simulink model "Depression"  (Simulink 6.3)
settings: Solver=ode23s  StartTime=0  StopTime=3500  MaxStep=0.5  RelTol=1e-3
undefined symbols (not defined in the file or in its folder): sigbuilder_block
Description:
  | This is a model of depression in synapses
settings Model: Creator=chchlee  LastModifiedBy=Owner  ExtModeAutoUpdateStatusClock=off
settings DataIOCC: SignalLoggingName=sigsOut
settings OptimizationCC: InlineInvariantSignals=on
settings DebuggingCC: SolverPrmCheckMsg=none
settings HardwareCC: TargetUnknown=on
settings GRTTargetCC: ModelReferenceCompliant=off  MatFileLogging=off

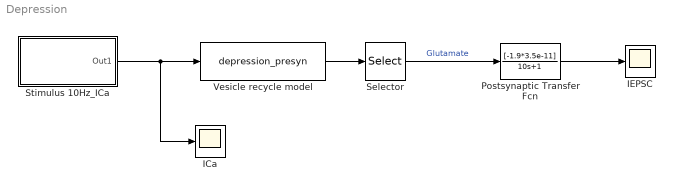
== system Depression ==
  ICa : Scope
      settings: YMin=-67.5  YMax=-63  SaveName=ScopeData3
  IEPSC : Scope
      settings: YMin=-2.2e-006  YMax=-1.04998e-038  SaveName=sim_depression10Hz  DataFormat=Array
  Postsynaptic Transfer Fcn : TransferFcn  Numerator=[-1.9*3.5e-11]  Denominator=[10 1]
  Selector : Selector  Elements=[4]  InputPortWidth=4
  Stimulus 10Hz_ICa : Subsystem
  Vesicle recycle model : S-Function  FunctionName=depression_presyn
  wires:
  Selector/1 -> Postsynaptic Transfer Fcn/1  "Glutamate"
  Vesicle recycle model/1 -> Selector/1
  Stimulus 10Hz_ICa/1(Out1) -> ICa/1, Vesicle recycle model/1
  Postsynaptic Transfer Fcn/1 -> IEPSC/1

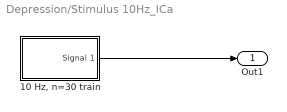
== system Depression/Stimulus 10Hz_ICa ==
  "10 Hz, n=30 train" : Subsystem  Tag=STV Subsys  LoadFcn=sigbuilder_block('load');  StartFcn=sigbuilder_block('start');  StopFcn=sigbuilder_block('stop');  ClipboardFcn=sigbuilder_block('clipboard');  mask(Sigbuilder block){}
      mask help: Sigbuilder GUI
      mask init:
      | if ~strcmp(get_param(bdroot(gcbh),'SimulationStatus'),'stopped') tuvar = sigbuilder_block('maskInit'); end
      settings: CopyFcn=sigbuilder_block('copy');  DeleteFcn=sigbuilder_block('delete');  ModelCloseFcn=sigbuilder_block('modelClose');  PreSaveFcn=sigbuilder_block('preSave');  NameChangeFcn=sigbuilder_block('namechange');  OpenFcn=sigbuilder_block('open',[-3 25.5 768 498 ]);  CloseFcn=sigbuilder_block('close');
      mask Display: plot(0,0,100,100,[10,10,40,40,10],[80,20,20,80,80],[40,10],[50,50], [40,27,10],[65,72,56],[40,25,25,10],[28,28,43,43]);
  Out1 : Outport
  wires:
  "10 Hz, n=30 train"/1(Signal 1) -> Out1/1

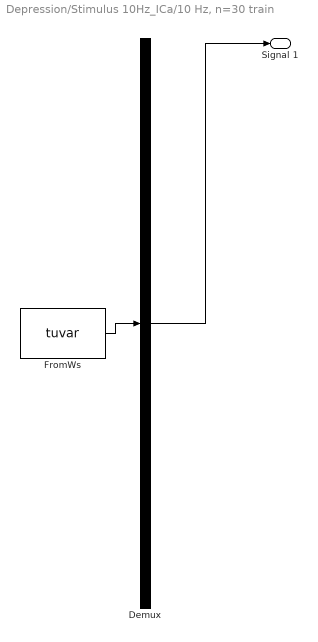
== system Depression/Stimulus 10Hz_ICa/10 Hz, n=30 train ==
  Demux : Demux  Tag=STV Demux  Outputs=1
  FromWs : FromWorkspace  Tag=STV FromWs  VariableName=tuvar  SampleTime=0  SigBuilderData=DataTag0  VnvData=DataTag1
      SigBuilderData=|
      | channels.label = 'Signal 1'
      | channels.allXData = {[0 100 100 101 101 200 200 201 201 300 300 301 301 400 400 401 401 500 500 501 501 600 600 601 601 700 700 701 701 800 800 801 801 900 900 901 901 1000 1000 1001 1001 1100 1100 1101 1101 1200 1200 1201 1201 1300 1300 1301 1301 1400 1400 1401 1401 1500 1500 1501 1501 1600 1600 1601 1601 1700 1700 1701 1701 1800 1800 1801 1801 1900 1900 1901 1901 2000 2000 2001 2001 2100 2100 2101 2101 2200 2200 2201 2201 2300 2300 2301 2301 2400 2400 2401 2401 2500 2500 2501 2501 2600 2600 2601 2601 2700 2700 2701 2701 2800 2800 2801 2801 2900 2900 2901 2901 3000 3000 3001 3001 3100 3100 3101 3101 3200 3300]}
      | channels.allYData = {[0 0 1 1 0 0 1 1 0 0 1 1 0 0 1 1 0 0 1 1 0 0 1 1 0 0 1 1 0 0 1 1 0 0 1 1 0 0 1 1 0 0 1 1 0 0 1 1 0 0 1 1 0 0 1 1 0 0 1 1 0 0 1 1 0 0 1 1 0 0 1 1 0 0 1 1 0 0 1 1 0 0 1 1 0 0 1 1 0 0 1 1 0 0 1 1 0 0 1 1 0 0 1 1 0 0 1 1 0 0 1 1 0 0 1 1 0 0 1 1 0 0 0 0 0 0 0]}
      | dataSet.timeRange = [0 3300]
      | dataSet.name = 'Group 1'
  Signal 1 : Outport  Tag=STV Outport
  wires:
  Demux/1 -> Signal 1/1
  FromWs/1 -> Demux/1
